simulink library "ArdupilotFunctions"  (R2024a)
settings: Solver=VariableStepAuto  StartTime=0.0  StopTime=10.0  RelTol=1e-3
undefined symbols (not defined in the file): DiscIntNeverNeededParam, gains, rates
libraries: eeGeneralControl x5
settings Model: Creator=igmso  LastModifiedBy=igmso

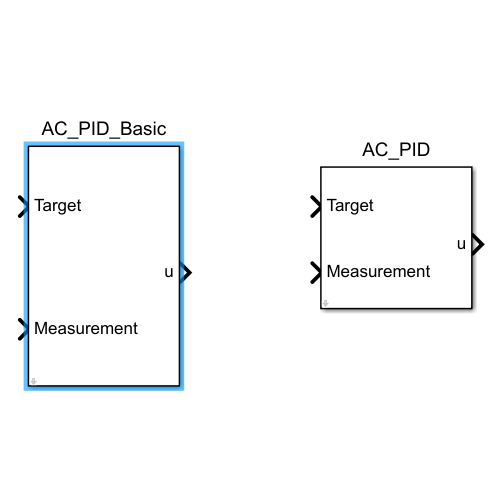
[thumbnail: Simulink's stored preview of the top-level diagram]
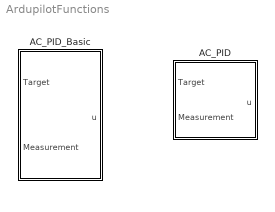
== system ArdupilotFunctions ==
  AC_PID : Subsystem  mask{P=gains.ACCZ_P, I=gains.ACCZ_I, D=0, FF=gains.ACCZ_FF*1e-3, D_FF=gains.ACCZ_D_FF*1e-3, FLTD=gains.ACCZ_FLTD, FLTE=gains.ACCZ_FLTE, FLTT=gains.ACCZ_FLTT, IMAX=gains.ACCZ_IMAX, ControlFreq=rates.PosControl}
      mask prompts: P "Proportional Gain:"; I "Integral Gain:"; D "Derivative Gain:"; FF "FeedForward Gain:"; D_FF "Derivative FeedForward Gain:"; FLTD "Controller Derivative Frequency in Hz:"; FLTE "Controller Error Frequency in Hz:"; FLTT "Controller Target Frequency in Hz:"; IMAX "Integral Gain Maximum:"; ControlFreq "Controlller Loop Rate:"
  AC_PID_Basic : Subsystem  mask{P=gains.VELZ_P, I=gains.VELZ_I, D=0, FF=gains.VELZ_FF, FLTD=50, FLTE=50, IMAX=gains.VELZ_IMAX, ControlFreq=rates.PosControl}
      mask prompts: P "Proportional Gain:"; I "Integral Gain:"; D "Derivative Gain:"; FF "FeedForward Gain :"; FLTD "Controller Derivative Frequency in Hz:"; FLTE "Controller Error Frequency in Hz:"; IMAX "Integral Gain Maximum:"; ControlFreq "Controller Loop Rate:"

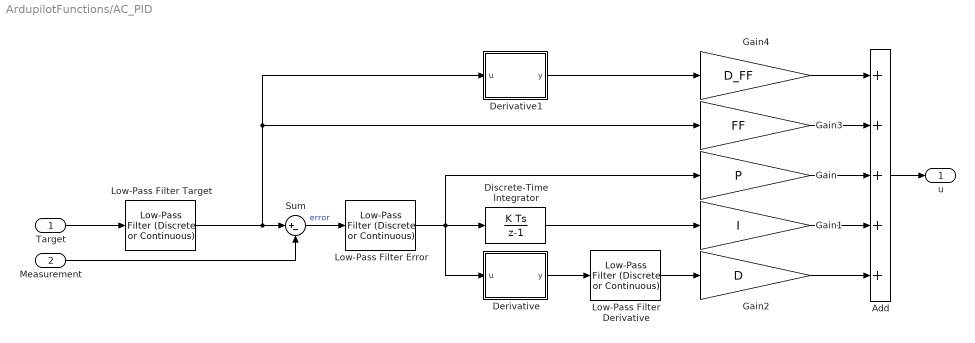
== system ArdupilotFunctions/AC_PID ==
  Target : Inport
  Measurement : Inport  Port=2
  Add : Sum  Inputs=5
  Derivative : Subsystem
  Derivative1 : Subsystem
  Discrete-Time Integrator : DiscreteIntegrator  SampleTime=-1  LimitOutput=on  UpperSaturationLimit=IMAX  LowerSaturationLimit=-IMAX  StateName='Accel_Z_I'  ICPrevOutput=DiscIntNeverNeededParam  ICPrevScaledInput=DiscIntNeverNeededParam
  Gain : Gain  Gain=P
  Gain1 : Gain  Gain=I
  Gain2 : Gain  Gain=D
  Gain3 : Gain  Gain=FF
  Gain4 : Gain  Gain=D_FF
  Low-Pass Filter Derivative : eeGeneralControl/Low-Pass Filter (Discrete or Continuous)  K=1  T=1/(2*pi*FLTD)  B=inf  A=-inf  init_option=Inherited from block input  x0=0  Ts=-1
  Low-Pass Filter Error : eeGeneralControl/Low-Pass Filter (Discrete or Continuous)  K=1  T=1/(2*pi*FLTE)  B=inf  A=-inf  init_option=Inherited from block input  x0=0  Ts=-1
  Low-Pass Filter Target : eeGeneralControl/Low-Pass Filter (Discrete or Continuous)  K=1  T=1/(2*pi*FLTT)  B=inf  A=-inf  init_option=Inherited from block input  x0=0  Ts=-1
  Sum : Sum  Inputs=|+-
  u : Outport
  wires:
  Derivative/1(y) -> Low-Pass Filter Derivative/1
  Low-Pass Filter Error/1 -> Discrete-Time Integrator/1, Gain/1, Derivative/1(u)
  Target/1 -> Low-Pass Filter Target/1
  Measurement/1 -> Sum/2
  Sum/1 -> Low-Pass Filter Error/1  "error"
  Discrete-Time Integrator/1 -> Gain1/1
  Low-Pass Filter Derivative/1 -> Gain2/1
  Gain/1 -> Add/3
  Gain1/1 -> Add/4
  Gain3/1 -> Add/2
  Gain2/1 -> Add/5
  Add/1 -> u/1
  Low-Pass Filter Target/1 -> Gain3/1, Derivative1/1(u), Sum/1
  Derivative1/1(y) -> Gain4/1
  Gain4/1 -> Add/1

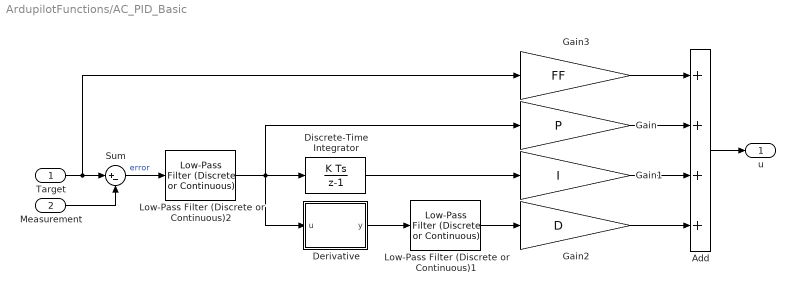
== system ArdupilotFunctions/AC_PID_Basic ==
  Target : Inport
  Measurement : Inport  Port=2
  Add : Sum  Inputs=4
  Derivative : Subsystem
  Discrete-Time Integrator : DiscreteIntegrator  SampleTime=-1  LimitOutput=on  UpperSaturationLimit=IMAX  LowerSaturationLimit=-IMAX  StateName='Vel_z_I'  ICPrevOutput=DiscIntNeverNeededParam  ICPrevScaledInput=DiscIntNeverNeededParam
  Gain : Gain  Gain=P
  Gain1 : Gain  Gain=I
  Gain2 : Gain  Gain=D
  Gain3 : Gain  Gain=FF
  Low-Pass Filter (Discrete or Continuous)1 : eeGeneralControl/Low-Pass Filter (Discrete or Continuous)  K=1  T=1/(2*pi*FLTD)  B=inf  A=-inf  init_option=Inherited from block input  x0=0  Ts=-1
  Low-Pass Filter (Discrete or Continuous)2 : eeGeneralControl/Low-Pass Filter (Discrete or Continuous)  K=1  T=1/(2*pi*FLTD)  B=inf  A=-inf  init_option=Inherited from block input  x0=0  Ts=-1
  Sum : Sum  Inputs=|+-
  u : Outport
  wires:
  Derivative/1(y) -> Low-Pass Filter (Discrete or Continuous)1/1
  Low-Pass Filter (Discrete or Continuous)2/1 -> Gain/1, Derivative/1(u), Discrete-Time Integrator/1
  Target/1 -> Gain3/1, Sum/1
  Measurement/1 -> Sum/2
  Sum/1 -> Low-Pass Filter (Discrete or Continuous)2/1  "error"
  Discrete-Time Integrator/1 -> Gain1/1
  Low-Pass Filter (Discrete or Continuous)1/1 -> Gain2/1
  Gain/1 -> Add/2
  Gain1/1 -> Add/3
  Gain3/1 -> Add/1
  Gain2/1 -> Add/4
  Add/1 -> u/1

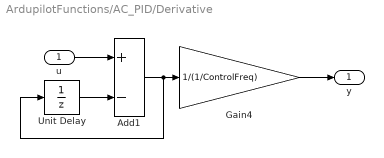
== system ArdupilotFunctions/AC_PID/Derivative ==
  u : Inport
  Add1 : Sum  Inputs=+-
  Gain4 : Gain  Gain=1/(1/ControlFreq)
  Unit Delay : UnitDelay  SampleTime=-1  HasFrameUpgradeWarning=on
  y : Outport
  wires:
  u/1 -> Add1/1
  Gain4/1 -> y/1
  Unit Delay/1 -> Add1/2
  Add1/1 -> Gain4/1, Unit Delay/1

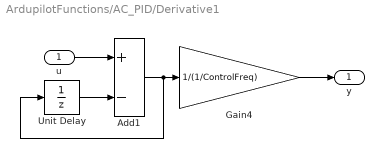
== system ArdupilotFunctions/AC_PID/Derivative1 ==
  u : Inport
  Add1 : Sum  Inputs=+-
  Gain4 : Gain  Gain=1/(1/ControlFreq)
  Unit Delay : UnitDelay  SampleTime=-1  HasFrameUpgradeWarning=on
  y : Outport
  wires:
  Add1/1 -> Unit Delay/1, Gain4/1
  Unit Delay/1 -> Add1/2
  Gain4/1 -> y/1
  u/1 -> Add1/1

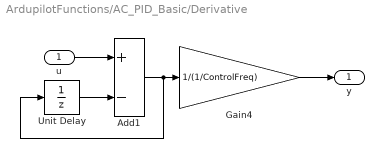
== system ArdupilotFunctions/AC_PID_Basic/Derivative ==
  u : Inport
  Add1 : Sum  Inputs=+-
  Gain4 : Gain  Gain=1/(1/ControlFreq)
  Unit Delay : UnitDelay  SampleTime=-1  HasFrameUpgradeWarning=on
  y : Outport
  wires:
  u/1 -> Add1/1
  Gain4/1 -> y/1
  Unit Delay/1 -> Add1/2
  Add1/1 -> Gain4/1, Unit Delay/1
